simulink model "vehicle_model_controller_ref"  (R2020b)
settings: Solver=VariableStepAuto  StartTime=0.0  StopTime=180  FixedStep=0.001  RelTol=1e-3
model workspace (MAT data in the model file):
  understeer_gradient = 0.05
undefined symbols (not defined in the file or in its folder): front_forces, rear_forces
libraries: fl_lib x24, nesl_utility x20, sdl_lib x8, autolibmappedmotor x4, vehdynlibsteering x1, pid_lib x1, autolibshared x1, autolibdatasheetbattery x1
(part 3 of 4)

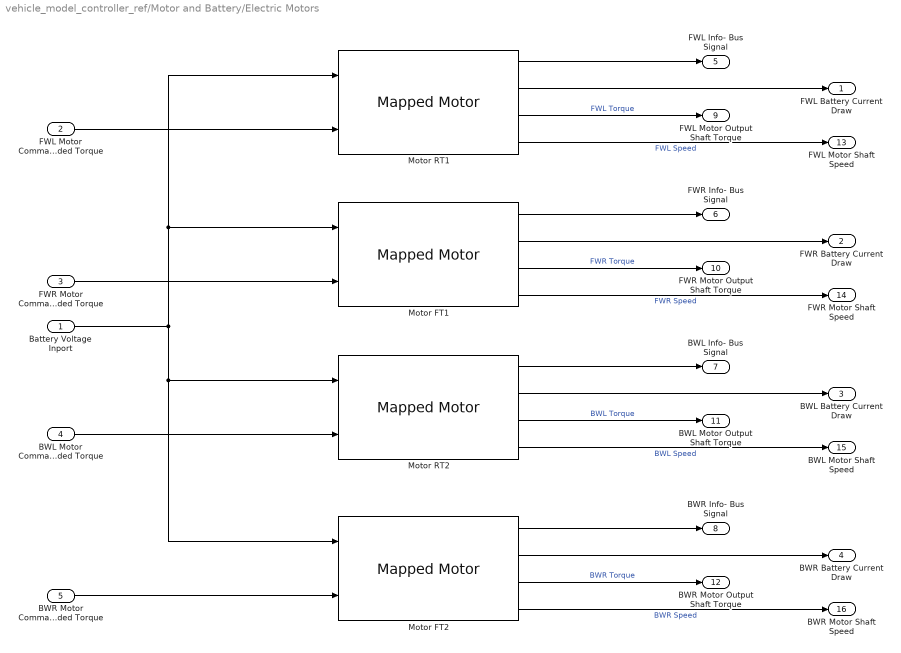
== system vehicle_model_controller_ref/Motor and Battery/Electric Motors ==
  Battery Voltage Inport : Inport
  FWL Motor Commanded Torque : Inport  Port=2
  "FWR Motor Commanded Torque " : Inport  Port=3
  BWL Motor Commanded Torque : Inport  Port=4
  BWR Motor Commanded Torque : Inport  Port=5
  Motor FT1 : autolibmappedmotor/Mapped Motor  port_config=Torque  param_by=Tabulated torque-speed envelope  w_t=[ 0 3750 7500 8000 11000]  T_t=[30 3 2 1 0.5]  torque_max=3  power_max=4000  Tc=0.02  param_loss=Single efficiency measurement  eff=100  w_eff=3750  T_eff=1.5  Piron=0  Pbase=0  w_eff_bp=[0 1000 2000 2728.370453 3000 4000 5000 6000 7000 8000 9000 10000]  T_eff_bp=[0 2 4 6 8 10 12 14 16 18 20 22 24 26 28]  Temp_eff_bp=[233.15 293.15 373.15]  losses_table=[1.49 1.67 2.21 3.10; 0.42 0.69 1.14 2.03; 0.06 0.24 0.78 1.68; 0.42 0.69 1.14 2.03; 1.49 1.67 2.21 3.10]  losses_table_3d=cat(3,1.05*[1.49 1.67 2.21 3.10; 0.42 0.69 1.14 2.03; 0.06 0.24 0.78 1.68; 0.42 0.69 1.14 2.03; 1.49 1.67 2.21 3.10],[1.49 1.67 2.21 3.10; 0.42 0.69 1.14 2.03; 0.06 0.24 0.78 1.68; 0.42 0.69 1.14 2.03; 1.49 1.67 2.21 3.10],1.03*[1.49 1.67 2.21 3.10; 0.42 0.69 1.14 2.03; 0.06 0.24 0.78 1.68; 0.42 0.69 1.14 2.03; 1.49 1.67 2.21 3.10])  efficiency_table=[85 85 85 85 85 85 85 85 85 85 85 85 85 85 85;85 85 85 85 85 85 85 85 85 85 85 85 85 85 85;85 85 90 90 90 90 90 90 90 90 88 88 88 88 88;85 85 92 92 92 92 92 92 92 92 92 90 90 90 90;85 85 92 92 93 93 93 93 92 92 92 90 90 90 90;85 85 93 94 94 94 94 94 94 94 94 94 94 94 94;85 85 93 94 94 95 95 95 95 95 95 95 95 95 95;85 85 93 94 94 95 95 95 95 95 95 95 95 95 95;85 85 93 94 95 95 95 95 95 95 95 95 95 95 95;85 85 93 94 95 95 95 95 95 95 95 95 95 95 95;85 85 93 94 94 94 94 94 94 94 94 94 94 94 94;85 85 90 92 93 93 93 93 93 93 93 93 93 93 93]  efficiency_table_3d=cat(3,90*ones(5,4),95*ones(5,4),92*ones(5,4))  J=5e-6  b=1e-5  omega_o=0  T_t_extended=[0.5 1 2 3 30 3 2 1 0.5]  w_t_extended=[-11000 -8000 -7500 -3750 0 3750 7500 8000 11000]  KLossIron=0  KLossCopper=0  x_w_eff_vec=[-10000 -9000 -8000 -7000 -6000 -5000 -4000 -3000 -2728.370453 -2000 -1000 0 1000 2000 2728.370453 3000 4000 5000 6000 7000 8000 9000 10000]  x_T_eff_vec=[-28 -26 -24 -22 -20 -18 -16 -14 -12 -10 -8 -6 -4 -2 0 2 4 6 8 10 12 14 16 18 20 22 24 26 28]  x_tmp_eff_vec=[233.15 293.15 373.15]  x_losses_mat=[21075.2688172043 19569.8924731183 18064.5161290322 16559.1397849462 15053.7634408602 13548.3870967742 12043.0107526882 10537.6344086021 9032.25806451612 7526.8817204301 6021.50537634408 5217.39130434782 4444.44444444445 3529.41176470588 0 3000 4000 4800 5600 7000 8399.99999999999 9799.99999999999 11200 12600 14000 15400 16800 18200 19600;16085.1063829787 14936.170212766 13787.2340425532 12638.2978723404 11489.3617021277 10340.4255319149 9191.48936170212 8042.55319148936 6893.61702127659 5744.68085106383 4595.74468085106 3446.8085106383 2709.67741935484 3176.47058823529 0 2700 2520 3240 4320 5399.99999999999 6479.99999999999 7559.99999999999 8639.99999999999 9719.99999999999 10800 11880 12960 14040 15120;11789.4736842105 10947.3684210526 10105.2631578947 9263.15789473683 8421.05263157894 7578.94736842104 6736.84210526315 5894.73684210526 5052.63157894736 4210.52631578947 3368.42105263158 3063.82978723404 2408.60215053763 2823.52941176471 0 2400 2240 2880 3200 3999.99999999999 4799.99999999999 5599.99999999999 6399.99999999999 7199.99999999999 7999.99999999999 8799.99999999999 9599.99999999999 10400 11200;10315.7894736842 9578.94736842104 8842.10526315788 8105.26315789473 7368.42105263157 6631.57894736841 5894.73684210526 5157.8947368421 4421.05263157894 3684.21052631579 2947.36842105263 2680.85106382979 2107.52688172043 2470.58823529412 0 2100 1960 2520 2800 3500 4199.99999999999 4899.99999999999 5599.99999999999 6299.99999999999 6999.99999999999 7699.99999999999 8399.99999999999 9099.99999999999 9799.99999999999;8842.10526315788 8210.52631578946 7578.94736842104 6947.36842105262 6315.7894736842 5684.21052631578 5052.63157894736 4421.05263157894 3789.47368421052 3157.8947368421 3063.82978723404 2297.87234042553 1806.45161290322 2117.64705882353 0 1800 1680 2160 2880 3000 3599.99999999999 4199.99999999999 4799.99999999999 5399.99999999999 5999.99999999999 6599.99999999999 7199.99999999999 7799.99999999999 8399.99999999999;7368.42105263157 6842.10526315789 6315.7894736842 5789.47368421052 5263.15789473684 4736.84210526315 4210.52631578947 3684.21052631579 3157.8947368421 2631.57894736842 2553.1914893617 1914.89361702128 1505.37634408602 1764.70588235294 0 1500 1400 1800 2400 2500 3000 3500 3999.99999999999 4499.99999999999 4999.99999999999 5499.99999999999 5999.99999999999 6499.99999999999 6999.99999999999;7148.93617021276 6638.29787234042 6127.65957446808 5617.02127659574 5106.3829787234 4595.74468085106 4085.10638297872 3574.46808510638 3063.82978723404 2553.1914893617 2042.55319148936 1531.91489361702 1204.30107526882 1411.76470588235 0 1200 1120 1440 1920 2400 2880 3360 3840 4320 4800 5279.99999999999 5759.99999999999 6239.99999999999 6719.99999999999;9333.33333333334 8666.66666666667 8000 7333.33333333334 5217.39130434782 4695.65217391304 4173.91304347826 3161.29032258064 2709.67741935484 2258.06451612903 1806.45161290322 1565.21739130435 1043.47826086956 1058.82352941176 0 900 960 1440 1680 2100 2520 2940 3840 4320 4800 6600 7200 7800 8400;8488.26363155556 7881.95908644445 7275.65454133334 6669.34999622222 4744.99209217391 4270.49288295652 3795.99367373913 3321.49446452174 2846.99525530435 2372.49604608695 1897.99683686956 1423.49762765217 948.998418434782 962.954277529412 0 818.5111359 873.07854496 1309.61781744 1746.15708992 2182.6963624 2619.23563488 3055.77490736 3492.31417984 3928.85345232 4365.3927248 6002.4149966 6548.0890872 7093.7631778 7639.4372684;7636.36363636364 7090.9090909091 6545.45454545455 6000 5454.54545454546 4000 3555.55555555556 3111.11111111111 2666.66666666667 2222.22222222222 1777.77777777778 1333.33333333333 888.888888888889 705.882352941177 0 600 800 1200 1600 2000 2400 2800 3200 3600 4800 5280 5760 6240 6720;4941.17647058824 4588.23529411765 4235.29411764706 3882.35294117647 3529.41176470588 3176.47058823529 2823.52941176471 2470.58823529412 2117.64705882353 1764.70588235294 1411.76470588235 1058.82352941176 705.882352941177 352.941176470588 0 300 600 900 1200 1500 1800 2100 2400 2700 3000 3300 ...(+4087 chars)]  x_losses_mat_3d=cat(3,[3.255 2.3205 1.7535 1.5645 1.7535 2.3205 3.255;2.1315 1.197 0.7245 0.441 0.7245 1.197 2.1315;1.764 0.819 0.252 0.063 0.252 0.819 1.764;2.1315 1.197 0.7245 0.441 0.7245 1.197 2.1315;3.255 2.3205 1.7535 1.5645 1.7535 2.3205 3.255],[3.1 2.21 1.67 1.49 1.67 2.21 3.1;2.03 1.14 0.69 0.42 0.69 1.14 2.03;1.68 0.78 0.24 0.06 0.24 0.78 1.68;2.03 1.14 0.69 0.42 0.69 1.14 2.03;3.1 2.21 1.67 1.49 1.67 2.21 3.1],[3.193 2.2763 1.7201 1.5347 1.7201 2.2763 3.193;2.0909 1.1742 0.7107 0.4326 0.7107 1.1742 2.0909;1.7304 0.8034 0.2472 0.0618 0.2472 0.8034 1.7304;2.0909 1.1742 0.7107 0.4326 0.7107 1.1742 2.0909;3.193 2.2763 1.7201 1.5347 1.7201 2.2763 3.193])  CalLossMapData={}  CalLossWithTempMapData={}  aMode=1  RefBlkName='autolibmappedmotor/Mapped Motor'
      settings: SourceProductBaseCode=PW,MT,UV,VE,VP
  Motor FT2 : autolibmappedmotor/Mapped Motor  port_config=Torque  param_by=Tabulated torque-speed envelope  w_t=[ 0 3750 7500 8000 11000]  T_t=[30 3 2 1 0.5]  torque_max=3  power_max=4000  Tc=0.02  param_loss=Tabulated efficiency data  eff=100  w_eff=3750  T_eff=1.5  Piron=0  Pbase=0  w_eff_bp=[0 1000 2000 2728.370453 3000 4000 5000 6000 7000 8000 9000 10000]  T_eff_bp=[0 2 4 6 8 10 12 14 16 18 20 22 24 26 28]  Temp_eff_bp=[233.15 293.15 373.15]  losses_table=[1.49 1.67 2.21 3.10; 0.42 0.69 1.14 2.03; 0.06 0.24 0.78 1.68; 0.42 0.69 1.14 2.03; 1.49 1.67 2.21 3.10]  losses_table_3d=cat(3,1.05*[1.49 1.67 2.21 3.10; 0.42 0.69 1.14 2.03; 0.06 0.24 0.78 1.68; 0.42 0.69 1.14 2.03; 1.49 1.67 2.21 3.10],[1.49 1.67 2.21 3.10; 0.42 0.69 1.14 2.03; 0.06 0.24 0.78 1.68; 0.42 0.69 1.14 2.03; 1.49 1.67 2.21 3.10],1.03*[1.49 1.67 2.21 3.10; 0.42 0.69 1.14 2.03; 0.06 0.24 0.78 1.68; 0.42 0.69 1.14 2.03; 1.49 1.67 2.21 3.10])  efficiency_table=[85 85 85 85 85 85 85 85 85 85 85 85 85 85 85;85 85 85 85 85 85 85 85 85 85 85 85 85 85 85;85 85 90 90 90 90 90 90 90 90 88 88 88 88 88;85 85 92 92 92 92 92 92 92 92 92 90 90 90 90;85 85 92 92 93 93 93 93 92 92 92 90 90 90 90;85 85 93 94 94 94 94 94 94 94 94 94 94 94 94;85 85 93 94 94 95 95 95 95 95 95 95 95 95 95;85 85 93 94 94 95 95 95 95 95 95 95 95 95 95;85 85 93 94 95 95 95 95 95 95 95 95 95 95 95;85 85 93 94 95 95 95 95 95 95 95 95 95 95 95;85 85 93 94 94 94 94 94 94 94 94 94 94 94 94;85 85 90 92 93 93 93 93 93 93 93 93 93 93 93]  efficiency_table_3d=cat(3,90*ones(5,4),95*ones(5,4),92*ones(5,4))  J=5e-6  b=1e-5  omega_o=0  T_t_extended=[0.5 1 2 3 30 3 2 1 0.5]  w_t_extended=[-11000 -8000 -7500 -3750 0 3750 7500 8000 11000]  KLossIron=0  KLossCopper=0  x_w_eff_vec=[-10000 -9000 -8000 -7000 -6000 -5000 -4000 -3000 -2728.370453 -2000 -1000 0 1000 2000 2728.370453 3000 4000 5000 6000 7000 8000 9000 10000]  x_T_eff_vec=[-28 -26 -24 -22 -20 -18 -16 -14 -12 -10 -8 -6 -4 -2 0 2 4 6 8 10 12 14 16 18 20 22 24 26 28]  x_tmp_eff_vec=[233.15 293.15 373.15]  x_losses_mat=[21075.2688172043 19569.8924731183 18064.5161290322 16559.1397849462 15053.7634408602 13548.3870967742 12043.0107526882 10537.6344086021 9032.25806451612 7526.8817204301 6021.50537634408 5217.39130434782 4444.44444444445 3529.41176470588 0 3000 4000 4800 5600 7000 8399.99999999999 9799.99999999999 11200 12600 14000 15400 16800 18200 19600;16085.1063829787 14936.170212766 13787.2340425532 12638.2978723404 11489.3617021277 10340.4255319149 9191.48936170212 8042.55319148936 6893.61702127659 5744.68085106383 4595.74468085106 3446.8085106383 2709.67741935484 3176.47058823529 0 2700 2520 3240 4320 5399.99999999999 6479.99999999999 7559.99999999999 8639.99999999999 9719.99999999999 10800 11880 12960 14040 15120;11789.4736842105 10947.3684210526 10105.2631578947 9263.15789473683 8421.05263157894 7578.94736842104 6736.84210526315 5894.73684210526 5052.63157894736 4210.52631578947 3368.42105263158 3063.82978723404 2408.60215053763 2823.52941176471 0 2400 2240 2880 3200 3999.99999999999 4799.99999999999 5599.99999999999 6399.99999999999 7199.99999999999 7999.99999999999 8799.99999999999 9599.99999999999 10400 11200;10315.7894736842 9578.94736842104 8842.10526315788 8105.26315789473 7368.42105263157 6631.57894736841 5894.73684210526 5157.8947368421 4421.05263157894 3684.21052631579 2947.36842105263 2680.85106382979 2107.52688172043 2470.58823529412 0 2100 1960 2520 2800 3500 4199.99999999999 4899.99999999999 5599.99999999999 6299.99999999999 6999.99999999999 7699.99999999999 8399.99999999999 9099.99999999999 9799.99999999999;8842.10526315788 8210.52631578946 7578.94736842104 6947.36842105262 6315.7894736842 5684.21052631578 5052.63157894736 4421.05263157894 3789.47368421052 3157.8947368421 3063.82978723404 2297.87234042553 1806.45161290322 2117.64705882353 0 1800 1680 2160 2880 3000 3599.99999999999 4199.99999999999 4799.99999999999 5399.99999999999 5999.99999999999 6599.99999999999 7199.99999999999 7799.99999999999 8399.99999999999;7368.42105263157 6842.10526315789 6315.7894736842 5789.47368421052 5263.15789473684 4736.84210526315 4210.52631578947 3684.21052631579 3157.8947368421 2631.57894736842 2553.1914893617 1914.89361702128 1505.37634408602 1764.70588235294 0 1500 1400 1800 2400 2500 3000 3500 3999.99999999999 4499.99999999999 4999.99999999999 5499.99999999999 5999.99999999999 6499.99999999999 6999.99999999999;7148.93617021276 6638.29787234042 6127.65957446808 5617.02127659574 5106.3829787234 4595.74468085106 4085.10638297872 3574.46808510638 3063.82978723404 2553.1914893617 2042.55319148936 1531.91489361702 1204.30107526882 1411.76470588235 0 1200 1120 1440 1920 2400 2880 3360 3840 4320 4800 5279.99999999999 5759.99999999999 6239.99999999999 6719.99999999999;9333.33333333334 8666.66666666667 8000 7333.33333333334 5217.39130434782 4695.65217391304 4173.91304347826 3161.29032258064 2709.67741935484 2258.06451612903 1806.45161290322 1565.21739130435 1043.47826086956 1058.82352941176 0 900 960 1440 1680 2100 2520 2940 3840 4320 4800 6600 7200 7800 8400;8488.26363155556 7881.95908644445 7275.65454133334 6669.34999622222 4744.99209217391 4270.49288295652 3795.99367373913 3321.49446452174 2846.99525530435 2372.49604608695 1897.99683686956 1423.49762765217 948.998418434782 962.954277529412 0 818.5111359 873.07854496 1309.61781744 1746.15708992 2182.6963624 2619.23563488 3055.77490736 3492.31417984 3928.85345232 4365.3927248 6002.4149966 6548.0890872 7093.7631778 7639.4372684;7636.36363636364 7090.9090909091 6545.45454545455 6000 5454.54545454546 4000 3555.55555555556 3111.11111111111 2666.66666666667 2222.22222222222 1777.77777777778 1333.33333333333 888.888888888889 705.882352941177 0 600 800 1200 1600 2000 2400 2800 3200 3600 4800 5280 5760 6240 6720;4941.17647058824 4588.23529411765 4235.29411764706 3882.35294117647 3529.41176470588 3176.47058823529 2823.52941176471 2470.58823529412 2117.64705882353 1764.70588235294 1411.76470588235 1058.82352941176 705.882352941177 352.941176470588 0 300 600 900 1200 1500 1800 2100 2400 2700 3000 3300 ...(+4087 chars)]  x_losses_mat_3d=cat(3,[3.255 2.3205 1.7535 1.5645 1.7535 2.3205 3.255;2.1315 1.197 0.7245 0.441 0.7245 1.197 2.1315;1.764 0.819 0.252 0.063 0.252 0.819 1.764;2.1315 1.197 0.7245 0.441 0.7245 1.197 2.1315;3.255 2.3205 1.7535 1.5645 1.7535 2.3205 3.255],[3.1 2.21 1.67 1.49 1.67 2.21 3.1;2.03 1.14 0.69 0.42 0.69 1.14 2.03;1.68 0.78 0.24 0.06 0.24 0.78 1.68;2.03 1.14 0.69 0.42 0.69 1.14 2.03;3.1 2.21 1.67 1.49 1.67 2.21 3.1],[3.193 2.2763 1.7201 1.5347 1.7201 2.2763 3.193;2.0909 1.1742 0.7107 0.4326 0.7107 1.1742 2.0909;1.7304 0.8034 0.2472 0.0618 0.2472 0.8034 1.7304;2.0909 1.1742 0.7107 0.4326 0.7107 1.1742 2.0909;3.193 2.2763 1.7201 1.5347 1.7201 2.2763 3.193])  CalLossMapData={}  CalLossWithTempMapData={}  aMode=1  RefBlkName='autolibmappedmotor/Mapped Motor'
      settings: SourceProductBaseCode=PW,MT,UV,VE,VP
  Motor RT1 : autolibmappedmotor/Mapped Motor  port_config=Torque  param_by=Tabulated torque-speed envelope  w_t=[ 0 3750 7500 8000 11000]  T_t=[30 3 2 1 0.5]  torque_max=3  power_max=4000  Tc=0.02  param_loss=Tabulated efficiency data  eff=100  w_eff=3750  T_eff=1.5  Piron=0  Pbase=0  w_eff_bp=[0 1000 2000 2728.370453 3000 4000 5000 6000 7000 8000 9000 10000]  T_eff_bp=[0 2 4 6 8 10 12 14 16 18 20 22 24 26 28]  Temp_eff_bp=[233.15 293.15 373.15]  losses_table=[1.49 1.67 2.21 3.10; 0.42 0.69 1.14 2.03; 0.06 0.24 0.78 1.68; 0.42 0.69 1.14 2.03; 1.49 1.67 2.21 3.10]  losses_table_3d=cat(3,1.05*[1.49 1.67 2.21 3.10; 0.42 0.69 1.14 2.03; 0.06 0.24 0.78 1.68; 0.42 0.69 1.14 2.03; 1.49 1.67 2.21 3.10],[1.49 1.67 2.21 3.10; 0.42 0.69 1.14 2.03; 0.06 0.24 0.78 1.68; 0.42 0.69 1.14 2.03; 1.49 1.67 2.21 3.10],1.03*[1.49 1.67 2.21 3.10; 0.42 0.69 1.14 2.03; 0.06 0.24 0.78 1.68; 0.42 0.69 1.14 2.03; 1.49 1.67 2.21 3.10])  efficiency_table=[85 85 85 85 85 85 85 85 85 85 85 85 85 85 85;85 85 85 85 85 85 85 85 85 85 85 85 85 85 85;85 85 90 90 90 90 90 90 90 90 88 88 88 88 88;85 85 92 92 92 92 92 92 92 92 92 90 90 90 90;85 85 92 92 93 93 93 93 92 92 92 90 90 90 90;85 85 93 94 94 94 94 94 94 94 94 94 94 94 94;85 85 93 94 94 95 95 95 95 95 95 95 95 95 95;85 85 93 94 94 95 95 95 95 95 95 95 95 95 95;85 85 93 94 95 95 95 95 95 95 95 95 95 95 95;85 85 93 94 95 95 95 95 95 95 95 95 95 95 95;85 85 93 94 94 94 94 94 94 94 94 94 94 94 94;85 85 90 92 93 93 93 93 93 93 93 93 93 93 93]  efficiency_table_3d=cat(3,90*ones(5,4),95*ones(5,4),92*ones(5,4))  J=5e-6  b=1e-5  omega_o=0  T_t_extended=[0.5 1 2 3 30 3 2 1 0.5]  w_t_extended=[-11000 -8000 -7500 -3750 0 3750 7500 8000 11000]  KLossIron=0  KLossCopper=0  x_w_eff_vec=[-10000 -9000 -8000 -7000 -6000 -5000 -4000 -3000 -2728.370453 -2000 -1000 0 1000 2000 2728.370453 3000 4000 5000 6000 7000 8000 9000 10000]  x_T_eff_vec=[-28 -26 -24 -22 -20 -18 -16 -14 -12 -10 -8 -6 -4 -2 0 2 4 6 8 10 12 14 16 18 20 22 24 26 28]  x_tmp_eff_vec=[233.15 293.15 373.15]  x_losses_mat=[21075.2688172043 19569.8924731183 18064.5161290322 16559.1397849462 15053.7634408602 13548.3870967742 12043.0107526882 10537.6344086021 9032.25806451612 7526.8817204301 6021.50537634408 5217.39130434782 4444.44444444445 3529.41176470588 0 3000 4000 4800 5600 7000 8399.99999999999 9799.99999999999 11200 12600 14000 15400 16800 18200 19600;16085.1063829787 14936.170212766 13787.2340425532 12638.2978723404 11489.3617021277 10340.4255319149 9191.48936170212 8042.55319148936 6893.61702127659 5744.68085106383 4595.74468085106 3446.8085106383 2709.67741935484 3176.47058823529 0 2700 2520 3240 4320 5399.99999999999 6479.99999999999 7559.99999999999 8639.99999999999 9719.99999999999 10800 11880 12960 14040 15120;11789.4736842105 10947.3684210526 10105.2631578947 9263.15789473683 8421.05263157894 7578.94736842104 6736.84210526315 5894.73684210526 5052.63157894736 4210.52631578947 3368.42105263158 3063.82978723404 2408.60215053763 2823.52941176471 0 2400 2240 2880 3200 3999.99999999999 4799.99999999999 5599.99999999999 6399.99999999999 7199.99999999999 7999.99999999999 8799.99999999999 9599.99999999999 10400 11200;10315.7894736842 9578.94736842104 8842.10526315788 8105.26315789473 7368.42105263157 6631.57894736841 5894.73684210526 5157.8947368421 4421.05263157894 3684.21052631579 2947.36842105263 2680.85106382979 2107.52688172043 2470.58823529412 0 2100 1960 2520 2800 3500 4199.99999999999 4899.99999999999 5599.99999999999 6299.99999999999 6999.99999999999 7699.99999999999 8399.99999999999 9099.99999999999 9799.99999999999;8842.10526315788 8210.52631578946 7578.94736842104 6947.36842105262 6315.7894736842 5684.21052631578 5052.63157894736 4421.05263157894 3789.47368421052 3157.8947368421 3063.82978723404 2297.87234042553 1806.45161290322 2117.64705882353 0 1800 1680 2160 2880 3000 3599.99999999999 4199.99999999999 4799.99999999999 5399.99999999999 5999.99999999999 6599.99999999999 7199.99999999999 7799.99999999999 8399.99999999999;7368.42105263157 6842.10526315789 6315.7894736842 5789.47368421052 5263.15789473684 4736.84210526315 4210.52631578947 3684.21052631579 3157.8947368421 2631.57894736842 2553.1914893617 1914.89361702128 1505.37634408602 1764.70588235294 0 1500 1400 1800 2400 2500 3000 3500 3999.99999999999 4499.99999999999 4999.99999999999 5499.99999999999 5999.99999999999 6499.99999999999 6999.99999999999;7148.93617021276 6638.29787234042 6127.65957446808 5617.02127659574 5106.3829787234 4595.74468085106 4085.10638297872 3574.46808510638 3063.82978723404 2553.1914893617 2042.55319148936 1531.91489361702 1204.30107526882 1411.76470588235 0 1200 1120 1440 1920 2400 2880 3360 3840 4320 4800 5279.99999999999 5759.99999999999 6239.99999999999 6719.99999999999;9333.33333333334 8666.66666666667 8000 7333.33333333334 5217.39130434782 4695.65217391304 4173.91304347826 3161.29032258064 2709.67741935484 2258.06451612903 1806.45161290322 1565.21739130435 1043.47826086956 1058.82352941176 0 900 960 1440 1680 2100 2520 2940 3840 4320 4800 6600 7200 7800 8400;8488.26363155556 7881.95908644445 7275.65454133334 6669.34999622222 4744.99209217391 4270.49288295652 3795.99367373913 3321.49446452174 2846.99525530435 2372.49604608695 1897.99683686956 1423.49762765217 948.998418434782 962.954277529412 0 818.5111359 873.07854496 1309.61781744 1746.15708992 2182.6963624 2619.23563488 3055.77490736 3492.31417984 3928.85345232 4365.3927248 6002.4149966 6548.0890872 7093.7631778 7639.4372684;7636.36363636364 7090.9090909091 6545.45454545455 6000 5454.54545454546 4000 3555.55555555556 3111.11111111111 2666.66666666667 2222.22222222222 1777.77777777778 1333.33333333333 888.888888888889 705.882352941177 0 600 800 1200 1600 2000 2400 2800 3200 3600 4800 5280 5760 6240 6720;4941.17647058824 4588.23529411765 4235.29411764706 3882.35294117647 3529.41176470588 3176.47058823529 2823.52941176471 2470.58823529412 2117.64705882353 1764.70588235294 1411.76470588235 1058.82352941176 705.882352941177 352.941176470588 0 300 600 900 1200 1500 1800 2100 2400 2700 3000 3300 ...(+4087 chars)]  x_losses_mat_3d=cat(3,[3.255 2.3205 1.7535 1.5645 1.7535 2.3205 3.255;2.1315 1.197 0.7245 0.441 0.7245 1.197 2.1315;1.764 0.819 0.252 0.063 0.252 0.819 1.764;2.1315 1.197 0.7245 0.441 0.7245 1.197 2.1315;3.255 2.3205 1.7535 1.5645 1.7535 2.3205 3.255],[3.1 2.21 1.67 1.49 1.67 2.21 3.1;2.03 1.14 0.69 0.42 0.69 1.14 2.03;1.68 0.78 0.24 0.06 0.24 0.78 1.68;2.03 1.14 0.69 0.42 0.69 1.14 2.03;3.1 2.21 1.67 1.49 1.67 2.21 3.1],[3.193 2.2763 1.7201 1.5347 1.7201 2.2763 3.193;2.0909 1.1742 0.7107 0.4326 0.7107 1.1742 2.0909;1.7304 0.8034 0.2472 0.0618 0.2472 0.8034 1.7304;2.0909 1.1742 0.7107 0.4326 0.7107 1.1742 2.0909;3.193 2.2763 1.7201 1.5347 1.7201 2.2763 3.193])  CalLossMapData={}  CalLossWithTempMapData={}  aMode=1  RefBlkName='autolibmappedmotor/Mapped Motor'
      settings: SourceProductBaseCode=PW,MT,UV,VE,VP
  Motor RT2 : autolibmappedmotor/Mapped Motor  port_config=Torque  param_by=Tabulated torque-speed envelope  w_t=[ 0 3750 7500 8000 11000]  T_t=[30 3 2 1 0.5]  torque_max=3  power_max=4000  Tc=0.02  param_loss=Tabulated efficiency data  eff=100  w_eff=3750  T_eff=1.5  Piron=0  Pbase=0  w_eff_bp=[0 1000 2000 2728.370453 3000 4000 5000 6000 7000 8000 9000 10000]  T_eff_bp=[0 2 4 6 8 10 12 14 16 18 20 22 24 26 28]  Temp_eff_bp=[233.15 293.15 373.15]  losses_table=[1.49 1.67 2.21 3.10; 0.42 0.69 1.14 2.03; 0.06 0.24 0.78 1.68; 0.42 0.69 1.14 2.03; 1.49 1.67 2.21 3.10]  losses_table_3d=cat(3,1.05*[1.49 1.67 2.21 3.10; 0.42 0.69 1.14 2.03; 0.06 0.24 0.78 1.68; 0.42 0.69 1.14 2.03; 1.49 1.67 2.21 3.10],[1.49 1.67 2.21 3.10; 0.42 0.69 1.14 2.03; 0.06 0.24 0.78 1.68; 0.42 0.69 1.14 2.03; 1.49 1.67 2.21 3.10],1.03*[1.49 1.67 2.21 3.10; 0.42 0.69 1.14 2.03; 0.06 0.24 0.78 1.68; 0.42 0.69 1.14 2.03; 1.49 1.67 2.21 3.10])  efficiency_table=[85 85 85 85 85 85 85 85 85 85 85 85 85 85 85;85 85 85 85 85 85 85 85 85 85 85 85 85 85 85;85 85 90 90 90 90 90 90 90 90 88 88 88 88 88;85 85 92 92 92 92 92 92 92 92 92 90 90 90 90;85 85 92 92 93 93 93 93 92 92 92 90 90 90 90;85 85 93 94 94 94 94 94 94 94 94 94 94 94 94;85 85 93 94 94 95 95 95 95 95 95 95 95 95 95;85 85 93 94 94 95 95 95 95 95 95 95 95 95 95;85 85 93 94 95 95 95 95 95 95 95 95 95 95 95;85 85 93 94 95 95 95 95 95 95 95 95 95 95 95;85 85 93 94 94 94 94 94 94 94 94 94 94 94 94;85 85 90 92 93 93 93 93 93 93 93 93 93 93 93]  efficiency_table_3d=cat(3,90*ones(5,4),95*ones(5,4),92*ones(5,4))  J=5e-6  b=1e-5  omega_o=0  T_t_extended=[0.5 1 2 3 30 3 2 1 0.5]  w_t_extended=[-11000 -8000 -7500 -3750 0 3750 7500 8000 11000]  KLossIron=0  KLossCopper=0  x_w_eff_vec=[-10000 -9000 -8000 -7000 -6000 -5000 -4000 -3000 -2728.370453 -2000 -1000 0 1000 2000 2728.370453 3000 4000 5000 6000 7000 8000 9000 10000]  x_T_eff_vec=[-28 -26 -24 -22 -20 -18 -16 -14 -12 -10 -8 -6 -4 -2 0 2 4 6 8 10 12 14 16 18 20 22 24 26 28]  x_tmp_eff_vec=[233.15 293.15 373.15]  x_losses_mat=[21075.2688172043 19569.8924731183 18064.5161290322 16559.1397849462 15053.7634408602 13548.3870967742 12043.0107526882 10537.6344086021 9032.25806451612 7526.8817204301 6021.50537634408 5217.39130434782 4444.44444444445 3529.41176470588 0 3000 4000 4800 5600 7000 8399.99999999999 9799.99999999999 11200 12600 14000 15400 16800 18200 19600;16085.1063829787 14936.170212766 13787.2340425532 12638.2978723404 11489.3617021277 10340.4255319149 9191.48936170212 8042.55319148936 6893.61702127659 5744.68085106383 4595.74468085106 3446.8085106383 2709.67741935484 3176.47058823529 0 2700 2520 3240 4320 5399.99999999999 6479.99999999999 7559.99999999999 8639.99999999999 9719.99999999999 10800 11880 12960 14040 15120;11789.4736842105 10947.3684210526 10105.2631578947 9263.15789473683 8421.05263157894 7578.94736842104 6736.84210526315 5894.73684210526 5052.63157894736 4210.52631578947 3368.42105263158 3063.82978723404 2408.60215053763 2823.52941176471 0 2400 2240 2880 3200 3999.99999999999 4799.99999999999 5599.99999999999 6399.99999999999 7199.99999999999 7999.99999999999 8799.99999999999 9599.99999999999 10400 11200;10315.7894736842 9578.94736842104 8842.10526315788 8105.26315789473 7368.42105263157 6631.57894736841 5894.73684210526 5157.8947368421 4421.05263157894 3684.21052631579 2947.36842105263 2680.85106382979 2107.52688172043 2470.58823529412 0 2100 1960 2520 2800 3500 4199.99999999999 4899.99999999999 5599.99999999999 6299.99999999999 6999.99999999999 7699.99999999999 8399.99999999999 9099.99999999999 9799.99999999999;8842.10526315788 8210.52631578946 7578.94736842104 6947.36842105262 6315.7894736842 5684.21052631578 5052.63157894736 4421.05263157894 3789.47368421052 3157.8947368421 3063.82978723404 2297.87234042553 1806.45161290322 2117.64705882353 0 1800 1680 2160 2880 3000 3599.99999999999 4199.99999999999 4799.99999999999 5399.99999999999 5999.99999999999 6599.99999999999 7199.99999999999 7799.99999999999 8399.99999999999;7368.42105263157 6842.10526315789 6315.7894736842 5789.47368421052 5263.15789473684 4736.84210526315 4210.52631578947 3684.21052631579 3157.8947368421 2631.57894736842 2553.1914893617 1914.89361702128 1505.37634408602 1764.70588235294 0 1500 1400 1800 2400 2500 3000 3500 3999.99999999999 4499.99999999999 4999.99999999999 5499.99999999999 5999.99999999999 6499.99999999999 6999.99999999999;7148.93617021276 6638.29787234042 6127.65957446808 5617.02127659574 5106.3829787234 4595.74468085106 4085.10638297872 3574.46808510638 3063.82978723404 2553.1914893617 2042.55319148936 1531.91489361702 1204.30107526882 1411.76470588235 0 1200 1120 1440 1920 2400 2880 3360 3840 4320 4800 5279.99999999999 5759.99999999999 6239.99999999999 6719.99999999999;9333.33333333334 8666.66666666667 8000 7333.33333333334 5217.39130434782 4695.65217391304 4173.91304347826 3161.29032258064 2709.67741935484 2258.06451612903 1806.45161290322 1565.21739130435 1043.47826086956 1058.82352941176 0 900 960 1440 1680 2100 2520 2940 3840 4320 4800 6600 7200 7800 8400;8488.26363155556 7881.95908644445 7275.65454133334 6669.34999622222 4744.99209217391 4270.49288295652 3795.99367373913 3321.49446452174 2846.99525530435 2372.49604608695 1897.99683686956 1423.49762765217 948.998418434782 962.954277529412 0 818.5111359 873.07854496 1309.61781744 1746.15708992 2182.6963624 2619.23563488 3055.77490736 3492.31417984 3928.85345232 4365.3927248 6002.4149966 6548.0890872 7093.7631778 7639.4372684;7636.36363636364 7090.9090909091 6545.45454545455 6000 5454.54545454546 4000 3555.55555555556 3111.11111111111 2666.66666666667 2222.22222222222 1777.77777777778 1333.33333333333 888.888888888889 705.882352941177 0 600 800 1200 1600 2000 2400 2800 3200 3600 4800 5280 5760 6240 6720;4941.17647058824 4588.23529411765 4235.29411764706 3882.35294117647 3529.41176470588 3176.47058823529 2823.52941176471 2470.58823529412 2117.64705882353 1764.70588235294 1411.76470588235 1058.82352941176 705.882352941177 352.941176470588 0 300 600 900 1200 1500 1800 2100 2400 2700 3000 3300 ...(+4087 chars)]  x_losses_mat_3d=cat(3,[3.255 2.3205 1.7535 1.5645 1.7535 2.3205 3.255;2.1315 1.197 0.7245 0.441 0.7245 1.197 2.1315;1.764 0.819 0.252 0.063 0.252 0.819 1.764;2.1315 1.197 0.7245 0.441 0.7245 1.197 2.1315;3.255 2.3205 1.7535 1.5645 1.7535 2.3205 3.255],[3.1 2.21 1.67 1.49 1.67 2.21 3.1;2.03 1.14 0.69 0.42 0.69 1.14 2.03;1.68 0.78 0.24 0.06 0.24 0.78 1.68;2.03 1.14 0.69 0.42 0.69 1.14 2.03;3.1 2.21 1.67 1.49 1.67 2.21 3.1],[3.193 2.2763 1.7201 1.5347 1.7201 2.2763 3.193;2.0909 1.1742 0.7107 0.4326 0.7107 1.1742 2.0909;1.7304 0.8034 0.2472 0.0618 0.2472 0.8034 1.7304;2.0909 1.1742 0.7107 0.4326 0.7107 1.1742 2.0909;3.193 2.2763 1.7201 1.5347 1.7201 2.2763 3.193])  CalLossMapData={}  CalLossWithTempMapData={}  aMode=1  RefBlkName='autolibmappedmotor/Mapped Motor'
      settings: SourceProductBaseCode=PW,MT,UV,VE,VP
  FWL Battery Current Draw : Outport
  FWR Battery Current Draw : Outport  Port=2
  BWL Battery Current Draw : Outport  Port=3
  BWR Battery Current Draw : Outport  Port=4
  FWL Info- Bus Signal : Outport  Port=5
  FWR Info- Bus Signal : Outport  Port=6
  BWL Info- Bus Signal : Outport  Port=7
  BWR Info- Bus Signal : Outport  Port=8
  FWL Motor Output Shaft Torque : Outport  Port=9
  FWR Motor Output Shaft Torque : Outport  Port=10
  BWL Motor Output Shaft Torque : Outport  Port=11
  BWR Motor Output Shaft Torque : Outport  Port=12
  FWL Motor Shaft Speed : Outport  Port=13
  FWR Motor Shaft Speed : Outport  Port=14
  BWL Motor Shaft Speed : Outport  Port=15
  BWR Motor Shaft Speed : Outport  Port=16
  wires:
  Motor FT2/3 -> BWR Motor Output Shaft Torque/1  "BWR Torque"
  Battery Voltage Inport/1 -> Motor FT2/1, Motor RT2/1, Motor FT1/1, Motor RT1/1
  Motor RT1/1 -> FWL Info- Bus Signal/1
  FWL Motor Commanded Torque/1 -> Motor RT1/2
  "FWR Motor Commanded Torque "/1 -> Motor FT1/2
  Motor RT2/1 -> BWL Info- Bus Signal/1
  Motor FT1/1 -> FWR Info- Bus Signal/1
  Motor FT2/1 -> BWR Info- Bus Signal/1
  Motor FT1/4 -> FWR Motor Shaft Speed/1  "FWR Speed"
  BWR Motor Commanded Torque/1 -> Motor FT2/2
  Motor RT2/4 -> BWL Motor Shaft Speed/1  "BWL Speed"
  Motor RT2/2 -> BWL Battery Current Draw/1
  Motor FT2/4 -> BWR Motor Shaft Speed/1  "BWR Speed"
  Motor FT2/2 -> BWR Battery Current Draw/1
  Motor RT1/3 -> FWL Motor Output Shaft Torque/1  "FWL Torque"
  BWL Motor Commanded Torque/1 -> Motor RT2/2
  Motor RT1/4 -> FWL Motor Shaft Speed/1  "FWL Speed"
  Motor FT1/3 -> FWR Motor Output Shaft Torque/1  "FWR Torque"
  Motor RT2/3 -> BWL Motor Output Shaft Torque/1  "BWL Torque"
  Motor RT1/2 -> FWL Battery Current Draw/1
  Motor FT1/2 -> FWR Battery Current Draw/1

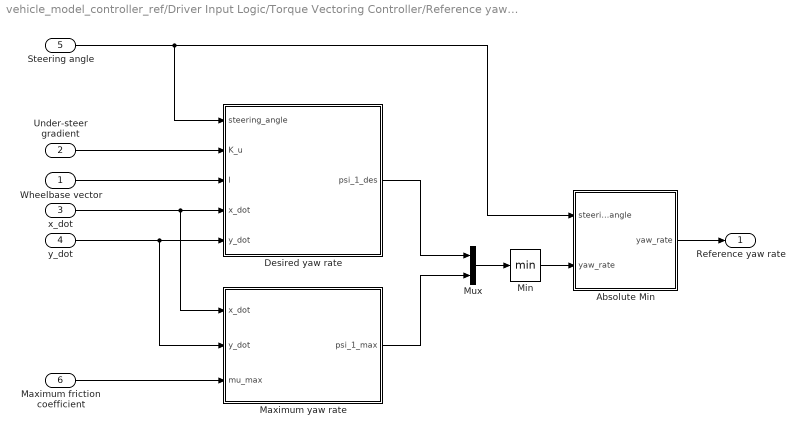
== system vehicle_model_controller_ref/Driver Input Logic/Torque Vectoring Controller/Reference yaw rate processor ==
  Wheelbase vector : Inport
  Under-steer gradient : Inport  Port=2
  x_dot : Inport  Port=3
  y_dot : Inport  Port=4
  "Steering angle " : Inport  Port=5
  Maximum friction coefficient : Inport  Port=6
  Absolute Min : MATLAB Function  TreatAsAtomicUnit=on
  Desired yaw rate : MATLAB Function  TreatAsAtomicUnit=on
  Maximum yaw rate : MATLAB Function  TreatAsAtomicUnit=on
  Min : MinMax
  Mux : Mux  Inputs=2
  Reference yaw rate : Outport
  wires:
  Wheelbase vector/1 -> Desired yaw rate/3(l)
  Under-steer gradient/1 -> Desired yaw rate/2(K_u)
  Absolute Min/1(yaw_rate) -> Reference yaw rate/1
  Maximum friction coefficient/1 -> Maximum yaw rate/3(mu_max)
  "Steering angle "/1 -> Desired yaw rate/1(steering_angle), Absolute Min/1(steering_angle)
  y_dot/1 -> Maximum yaw rate/2(y_dot), Desired yaw rate/5(y_dot)
  x_dot/1 -> Desired yaw rate/4(x_dot), Maximum yaw rate/1(x_dot)
  Mux/1 -> Min/1
  Desired yaw rate/1(psi_1_des) -> Mux/1
  Maximum yaw rate/1(psi_1_max) -> Mux/2
  Min/1 -> Absolute Min/2("yaw_rate ")

== system vehicle_model_controller_ref/Electric Vehicle Model/Vehicle Body/Mechanical Braking Effects ==
  motor_force : Inport
  braking_	force : Inport  Port=2
  Bus Selector : BusSelector  OutputSignals=front_forces,rear_forces
  mechanical_braking_effects : MATLAB Function  TreatAsAtomicUnit=on
  FwF : Outport
  FwR : Outport  Port=2
  wires:
  mechanical_braking_effects/1(FwF) -> FwF/1
  braking_	force/1 -> mechanical_braking_effects/1(braking_forces)
  mechanical_braking_effects/2(FwR) -> FwR/1
  Bus Selector/1 -> mechanical_braking_effects/2(front_forces)  "<front_forces>"
  Bus Selector/2 -> mechanical_braking_effects/3(rear_forces)  "<rear_forces>"
  motor_force/1 -> Bus Selector/1

== matlab function vehicle_model_controller_ref/Electric Vehicle Model/Vehicle Body/Mechanical Braking Effects/mechanical_braking_effects ==
  data: braking_forces input; front_forces input; FwF output; rear_forces input; FwR output
function [FwF, FwR] = Mechanical_Braking_Effects(braking_forces, front_forces, rear_forces)
%% Mechanical Braking Effects
% Developers:    Demetrius Gulewicz
% Developed for: Purdue Electric Racing
% Date:          09/01/2021
%
% Definitions:
% front_force:      force vector from the front motors    [N]
% braking_forces:   braking force vector on all 4 tires   [N]
% rear_forces:      force vector from the rear motors     [N]

%% Calculation
FwF = front_forces - braking_forces(1:2);
FwR = rear_forces - braking_forces(3:4);

== matlab function vehicle_model_controller_ref/Driver Input Logic/Torque Vectoring Controller/Reference yaw rate processor/Absolute Min ==
  data: steering_angle input; yaw_rate output; yaw_rate input
function yaw_rate = absolute_min(steering_angle, yaw_rate)
if steering_angle >= 0 % this part is to judge the direction of yaw,
    i = 1;
else
    i = -1;
end
yaw_rate = i * yaw_rate;
